simulink model "Nonlinear"  (R2019b)
settings: Solver=VariableStepAuto  StartTime=0.0  StopTime=10  FixedStep=0.1  RelTol=1e-3
settings Model: Creator=miaokeyan  LastModifiedBy=miaokeyan
settings SolverCC: ShapePreserveControl=EnableAll  ZeroCrossControl=DisableAll
settings DataIOCC: ReturnWorkspaceOutputs=off
settings DebuggingCC: ArithmeticOperatorsInVariantConditions=warning
settings SFSimCC: SimUseLocalCustomCode=off  CustomCodeUndefinedFunction=UseInterfaceOnly
settings RTWCC: RTWUseLocalCustomCode=off
settings CodeAppCC: StateflowObjectComments=on

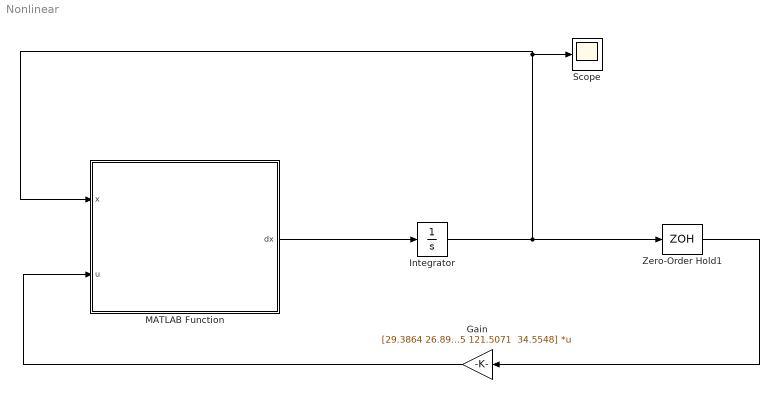
== system Nonlinear ==
  Gain : Gain  Gain="[29.3864 26.8975 121.5071  34.5548]"  Multiplication=Matrix(K*u) (u vector)
  Integrator : Integrator  InitialCondition=[0 0.1 0.6 1]
  MATLAB Function : MATLAB Function  TreatAsAtomicUnit=on
  Scope : Scope
  Zero-Order Hold1 : ZeroOrderHold  SampleTime=0.001
  wires:
  MATLAB Function/1(dx) -> Integrator/1
  Integrator/1 -> Zero-Order Hold1/1, MATLAB Function/1(x), Scope/1
  Zero-Order Hold1/1 -> Gain/1
  Gain/1 -> MATLAB Function/2(u)

== matlab function Nonlinear/MATLAB Function ==
  data: x input; dx output; u input
function dx = fcn(x,u)
F = 1;
M = 1;
L = 0.842;
g = 9.8093;
dx = zeros(4,1);
% K = [103.0043  112.5880  687.6229  137.7411];
% u = K * [x1; x2; x3; x4];

dx(1) = x(2);
dx(2) = -F*x(2)/M + u/M;
dx(3) = x(4);
dx(4) = F*cos(x(3))*x(2)/(L*M) + g*sin(x(3))/L - cos(x(3))*u/(L*M);
